simulink model "SiC_Mosfet_model_2"  (R2019b)
settings: Solver=VariableStepAuto  StartTime=0.0  StopTime=10.0  RelTol=1e-3
values from neighbouring files (symbols this model uses):
  T = etemp_input    [etemp_function.m]    (also in ftemp_function.m = ftemp_input)
  Vds = core_inputs(2)    [core_function.m]    (also in core_funtion.m)
  Vgs = core_inputs(1)    [core_function.m]    (also in core_funtion.m)
libraries: nesl_utility x9, ee_lib x7, fl_lib x3
settings Model: Creator=karth  LastModifiedBy=Anoop
settings SFSimCC: CustomCodeUndefinedFunction=UseInterfaceOnly

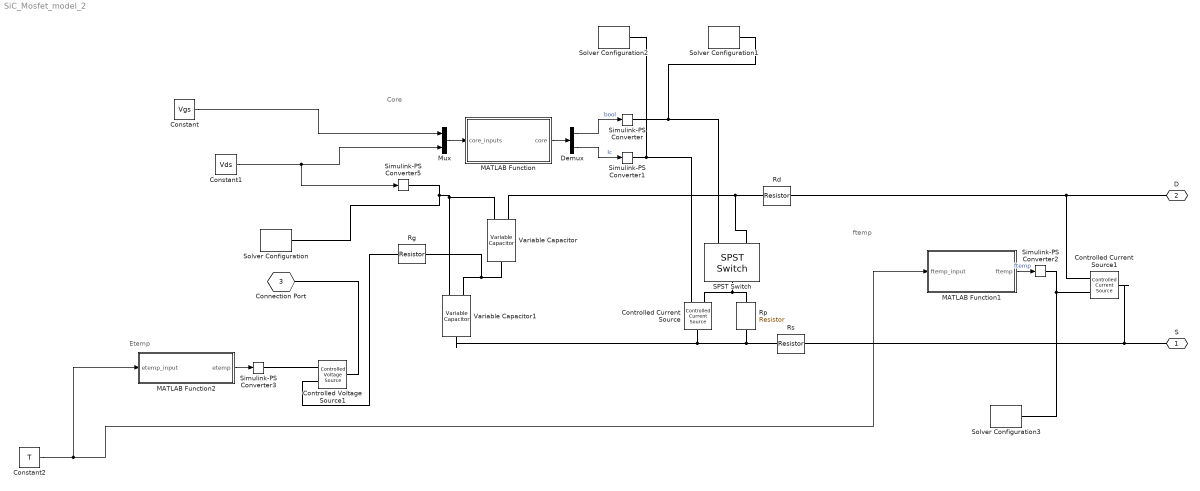
== system SiC_Mosfet_model_2 ==
  note: Etemp
  note: ftemp
  note: Core
  Constant : Constant  Value=Vgs
  Constant1 : Constant  Value=Vds
  Constant2 : Constant  Value=T
  Controlled Current Source : fl_lib/Electrical/Electrical Sources/Controlled Current Source
  Controlled Current Source1 : fl_lib/Electrical/Electrical Sources/Controlled Current Source
  Controlled Voltage Source1 : fl_lib/Electrical/Electrical Sources/Controlled Voltage Source
  Demux : Demux  Outputs=2
  MATLAB Function : MATLAB Function  TreatAsAtomicUnit=on
  MATLAB Function1 : MATLAB Function  TreatAsAtomicUnit=on
  MATLAB Function2 : MATLAB Function  TreatAsAtomicUnit=on
  Mux : Mux  Inputs=2
  Rd : ee_lib/Passive/Resistor  R=1 Ohm  R_tol=5  enable_R_tol=0  tol_distribution=1  nSigma=4  enable_operating_limits=0  operating_limit_action=2  max_working_voltage=100 V  power_rating=1 W  enable_faults=0  fault_action=1  R_faulted=inf Ohm  enable_temporal_fault=0  t_fault=1 s  enable_behavioral_fault=0  max_permissible_current=1 A  t_fail_on_current=1 s  noise_mode=0  sample_time=1e-3 s  repeatability=1  auto_seed=2715962282  user_seed=0  Tdevice=25 degC  alpha=3.93e-3 1/K  Tmeas=25 degC  thermal_mass=100 J/K  power_derating_T1=70 degC  power_derating_T2=155 degC  operating_temperature_range_vec=[-50, 150] degC  temperature_specify=off  temperature_priority=High  temperature=298.15 K  temperature_nominal_specify=off  temperature_nominal_unit=K  temperature_nominal_value=1
      settings: SourceProductName=Simscape Electrical
  Rg : ee_lib/Passive/Resistor  R=1 Ohm  R_tol=5  enable_R_tol=0  tol_distribution=1  nSigma=4  enable_operating_limits=0  operating_limit_action=2  max_working_voltage=100 V  power_rating=1 W  enable_faults=0  fault_action=1  R_faulted=inf Ohm  enable_temporal_fault=0  t_fault=1 s  enable_behavioral_fault=0  max_permissible_current=1 A  t_fail_on_current=1 s  noise_mode=0  sample_time=1e-3 s  repeatability=1  auto_seed=418932850  user_seed=0  Tdevice=25 degC  alpha=3.93e-3 1/K  Tmeas=25 degC  thermal_mass=100 J/K  power_derating_T1=70 degC  power_derating_T2=155 degC  operating_temperature_range_vec=[-50, 150] degC  temperature_specify=off  temperature_priority=High  temperature=298.15 K  temperature_nominal_specify=off  temperature_nominal_unit=K  temperature_nominal_value=1
      settings: SourceProductName=Simscape Electrical
  Rp : ee_lib/Passive/Resistor  R=1 Ohm  R_tol=5  enable_R_tol=0  tol_distribution=1  nSigma=4  enable_operating_limits=0  operating_limit_action=2  max_working_voltage=100 V  power_rating=1 W  enable_faults=0  fault_action=1  R_faulted=inf Ohm  enable_temporal_fault=0  t_fault=1 s  enable_behavioral_fault=0  max_permissible_current=1 A  t_fail_on_current=1 s  noise_mode=0  sample_time=1e-3 s  repeatability=1  auto_seed=1196140742  user_seed=0  Tdevice=25 degC  alpha=3.93e-3 1/K  Tmeas=25 degC  thermal_mass=100 J/K  power_derating_T1=70 degC  power_derating_T2=155 degC  operating_temperature_range_vec=[-50, 150] degC  temperature_specify=off  temperature_priority=High  temperature=298.15 K  temperature_nominal_specify=off  temperature_nominal_unit=K  temperature_nominal_value=1
      settings: SourceProductName=Simscape Electrical
  Rs : ee_lib/Passive/Resistor  R=1 Ohm  R_tol=5  enable_R_tol=0  tol_distribution=1  nSigma=4  enable_operating_limits=0  operating_limit_action=2  max_working_voltage=100 V  power_rating=1 W  enable_faults=0  fault_action=1  R_faulted=inf Ohm  enable_temporal_fault=0  t_fault=1 s  enable_behavioral_fault=0  max_permissible_current=1 A  t_fail_on_current=1 s  noise_mode=0  sample_time=1e-3 s  repeatability=1  auto_seed=2348838240  user_seed=0  Tdevice=25 degC  alpha=3.93e-3 1/K  Tmeas=25 degC  thermal_mass=100 J/K  power_derating_T1=70 degC  power_derating_T2=155 degC  operating_temperature_range_vec=[-50, 150] degC  temperature_specify=off  temperature_priority=High  temperature=298.15 K  temperature_nominal_specify=off  temperature_nominal_unit=K  temperature_nominal_value=1
      settings: SourceProductName=Simscape Electrical
  SPST Switch : ee_lib/Switches & Breakers/SPST Switch  R_closed=0.01 Ohm  G_open=1e-6 S  Threshold=0.5 V  Width=0 V  model_dynamics=0  t_on=1e-3 s  t_off=1e-3 s  initial_vT=0 V
      settings: SourceProductName=Simscape Electrical  SourceProductBaseCode=PS  InternalSimscapePortConfiguration="{\"Bottom\":[],\"Left\":[{\"id\":\"vT\",\"label\":\"vT\",\"type\":\"input\"},{\"id\":\"p\",\"label\":\"\",\"type\":\"foundation.electrical.electrical\"}],\"Right\":[{\"id\":\"n\",\"label\":\"\",\"type\":\"foundation.electrical.electrical\"}],\"Top\":[]}"
  Simulink-PS Converter{,1..3,5} (5 alike) : nesl_utility/Simulink-PS Converter  PhysicalDomain=network_engine_domain  SubClassName=ps_input  LeftPortType=input  RightPortType=output  PseudoPeriodic=off  Frequencies=[]  NoiseDistribution=none  NoiseParameters=[]  Unit=1  AffineConversion=off  FilteringAndDerivatives=provide  SimscapeFilterOrder=1  InputFilterTimeConstant=0.001  UdotUserProvided=0
  Solver Configuration{,1..3} (4 alike) : nesl_utility/Solver Configuration  PhysicalDomain=network_engine_domain  SubClassName=solver  LeftPortType=input  RightPortType=generic  Tones=[]  Harmonics=[]  SimulateNoise=off  Profile=off  UseLocalSampling=off  EnableSwitchedLinearOptims=on  FrequencyDomain=off  UseCCode=off  RelTol=0.001  AbsTol=1e-06  MinStep=1e-09  ToWorkspace=off  RevertToSquareIcSolve=off  NumHomotopyIterations=100  PhasorMode=off  PhasorModeNumHarmonics=1  DoDC=off  ResidualTolerance=1e-09  UseLocalSolver=off  LocalSolverChoice=NE_BACKWARD_EULER_ADVANCER  LocalSolverSampleTime=0.001  DoFixedCost=off  MaxNonlinIter=3  MaxModeIter=2  LinearAlgebra=auto  EquationFormulation=NE_TIME_EF  DelaysMemoryBudget=1024  AutomaticFiltering=on  FilteringTimeConstant=0.001  PartitionStorageMethod=AS_NEEDED  PartitionMemoryBudget=1024  PartitionMethod=ROBUST
  Variable Capacitor : ee_lib/Passive/Variable Capacitor  prm=2  Cmin=1e-9 F  r=1e-6 Ohm  v0=0 V  q0=0 C
      settings: SourceProductName=Simscape Electrical  SourceProductBaseCode=PS  InternalSimscapePortConfiguration="{\"Bottom\":[],\"Left\":[{\"id\":\"C\",\"label\":\"C\",\"type\":\"input\"},{\"id\":\"p\",\"label\":\"+\",\"type\":\"foundation.electrical.electrical\"}],\"Right\":[{\"id\":\"n\",\"label\":\"-\",\"type\":\"foundation.electrical.electrical\"}],\"Top\":[]}"
  Variable Capacitor1 : ee_lib/Passive/Variable Capacitor  prm=2  Cmin=1e-9 F  r=1e-6 Ohm  v0=0 V  q0=0 C
      settings: SourceProductName=Simscape Electrical  SourceProductBaseCode=PS  InternalSimscapePortConfiguration="{\"Bottom\":[],\"Left\":[{\"id\":\"C\",\"label\":\"C\",\"type\":\"input\"},{\"id\":\"p\",\"label\":\"+\",\"type\":\"foundation.electrical.electrical\"}],\"Right\":[{\"id\":\"n\",\"label\":\"-\",\"type\":\"foundation.electrical.electrical\"}],\"Top\":[]}"
  S : PMIOPort  Side=Left
  D : PMIOPort  Port=2  Side=Left
  Connection Port : PMIOPort  Tag=PMCPort  Port=3  Side=Left
  wires:
  Demux/1 -> Simulink-PS Converter/1  "bool"
  Demux/2 -> Simulink-PS Converter1/1  "Ic"
  Constant/1 -> Mux/1
  Constant2/1 -> MATLAB Function2/1(etemp_input), MATLAB Function1/1(ftemp_input)
  Mux/1 -> MATLAB Function/1(core_inputs)
  MATLAB Function/1(core) -> Demux/1
  MATLAB Function1/1(ftemp) -> Simulink-PS Converter2/1  "ftemp"
  MATLAB Function2/1(etemp) -> Simulink-PS Converter3/1
  Constant1/1 -> Simulink-PS Converter5/1, Mux/2
  connections:
  Rs/LConn1 -- Controlled Current Source1/LConn1 -- S/RConn1
  Rd/LConn1 -- Controlled Current Source1/RConn2 -- D/RConn1
  Simulink-PS Converter/RConn1 -- SPST Switch/LConn1 -- Solver Configuration1/RConn1
  Simulink-PS Converter1/RConn1 -- Solver Configuration2/RConn1 -- Controlled Current Source/RConn1
  SPST Switch/RConn1 -- Controlled Current Source/RConn2 -- Rp/LConn1
  Rd/RConn1 -- Variable Capacitor/LConn2 -- SPST Switch/LConn2
  Rp/RConn1 -- Rs/RConn1 -- Controlled Current Source/LConn1 -- Variable Capacitor1/RConn1
  Simulink-PS Converter2/RConn1 -- Solver Configuration3/RConn1 -- Controlled Current Source1/RConn1
  Simulink-PS Converter5/RConn1 -- Solver Configuration/RConn1 -- Variable Capacitor1/LConn1 -- Variable Capacitor/LConn1
  Variable Capacitor/RConn1 -- Rg/LConn1 -- Variable Capacitor1/LConn2
  Controlled Voltage Source1/RConn1 -- Simulink-PS Converter3/RConn1
  Controlled Voltage Source1/RConn2 -- Rg/RConn1
  Connection Port/RConn1 -- Controlled Voltage Source1/LConn1

== matlab function SiC_Mosfet_model_2/MATLAB Function1 ==
  data: ftemp_input input; ftemp output
%%%%%%%%%%%%%%%%%%%%%%%%%%%%%%%%%%%%%%%%%%%%%%%%%%%%%%%%%%%%%%%%%%%%%%%%%%%
% File name: ftemp_function.m
% Authors: Karthik K Bhat, Anoop Narayana, Maithili Shetty
%%%%%%%%%%%%%%%%%%%%%%%%%%%%%%%%%%%%%%%%%%%%%%%%%%%%%%%%%%%%%%%%%%%%%%%%%%%

function ftemp = ftemp_function(ftemp_input)    
    T = ftemp_inputs(1);
    ftemp = Idstd*(((Tstd/T)^K_temp));
end

== matlab function SiC_Mosfet_model_2/MATLAB Function ==
  data: core_inputs input; core output
%%%%%%%%%%%%%%%%%%%%%%%%%%%%%%%%%%%%%%%%%%%%%%%%%%%%%%%%%%%%%%%%%%%%%%%%%%%
% File name: core_function.m
% Authors: Karthik K Bhat, Anoop Narayana, Maithili Shetty 
%%%%%%%%%%%%%%%%%%%%%%%%%%%%%%%%%%%%%%%%%%%%%%%%%%%%%%%%%%%%%%%%%%%%%%%%%%%

% ----------------------------------------------------------------------- %

function core = core_funtion(core_inputs)
    Vgs = core_inputs(1);
    Vds = core_inputs(2);
    if (Vgs < Vth)
        Id = 0;
    elseif ((Vds > 0) && (Vds < ((Vgs - Vth)/(1+a))))
        Id = k * (((Vgs-Vth)*Vds) - (((1+a)*Vds^2)/2))*(1+lambda*Vds);
    elseif ((Vds > (Vgs-Vth)/(1+a)) &&  ((Vgs-Vth)/(1+a) > 0))
        Id = (k / 2*(1+a)) * (1+lambda*Vds) * (Vgs - Vth)^2;
    end
core = Id;
end

    function y = fcn(u)

y = u;

== matlab function SiC_Mosfet_model_2/MATLAB Function2 ==
  data: etemp_input input; etemp output
%%%%%%%%%%%%%%%%%%%%%%%%%%%%%%%%%%%%%%%%%%%%%%%%%%%%%%%%%%%%%%%%%%%%%%%%%%%
% File name: etemp_function.m
% Authors: Karthik K Bhat, Anoop Narayana, Maithili Shetty
%%%%%%%%%%%%%%%%%%%%%%%%%%%%%%%%%%%%%%%%%%%%%%%%%%%%%%%%%%%%%%%%%%%%%%%%%%%

function etemp = etemp_function(etemp_input)
    global Tstd alpha
    T = etemp_input;   
    etemp = (T - Tstd) * alpha;
end  function y = fcn(u)

y = u;
